simulink model "Nerthus_sim"  (R2021a)
settings: Solver=ode45  StartTime=0.0  StopTime=simtime  MaxStep=ts_max
values from neighbouring files (symbols this model uses):
  a_f = 1E-5*depl_fuel_temp_coef(depl_index)    [parameters.m]
  a_g = 1E-5*depl_grap_temp_coef(depl_index)    [parameters.m]
  A_s = 1.2245    [parameters.m]
  beta = depl_beta(depl_index,:)    [parameters.m]
  beta_t = sum(beta)    [parameters.m]
  Cp_1 = mean(interp1(Cal_temp1, Cal_Cp1, region_fdw))/1e3    [parameters.m]
  Cp_2 = mean(interp1(Cal_temp2, Cal_Cp2, region_sc))/1e3    [parameters.m]
  Cp_3 = mean(interp1(Cal_temp3, Cal_Cp3, region_s2))/1e3    [parameters.m]
  Cp_4 = mean(interp1(Cal_temp4, Cal_Cp4, region_s1))/1e3    [parameters.m]
  Cp_p = 0.00154912    [parameters.m]
  Cp_w = 456.056e-6    (= 0.000456056)    [parameters.m]
  D_it = 0.0141478    [parameters.m]
  D_ot = 0.015875    [parameters.m]
  DHRS_MODE = 1    [parameters.m]    (also in transients.m)
  DHRS_Power = P*(0.10)    (= 55.7)    [parameters.m]    (also in transients.m)
  DHRS_time = 20000000    [parameters.m]    (also in transients.m)
  DHRS_TIME_K = 10    [parameters.m]
  dHs_dPs = -0.042433622114357    (= -0.0424336221144)    [parameters.m]
  Epsilon = 1E-3    (= 0.001)    [parameters.m]
  Fiss_factor = 2.464783802008740e-03    (= 0.00246478380201)    [parameters.m]
  gamma0 = 9.635981959409105e-01    (= 0.963598195941)    [parameters.m]
  gamma1 = 3.560674858154914e-02    (= 0.0356067485815)    [parameters.m]
  gamma2 = 7.950554775404400e-04    (= 0.00079505547754)    [parameters.m]
  gamma_I = 5.1135e-2    (= 0.051135)    [parameters.m]
  gamma_Te = 6.1e-2    (= 0.061)    [parameters.m]
  gamma_Xe = 1.1628e-2    (= 0.011628)    [parameters.m]
  h_pw = h_s_shx    (= 0.00910134357894)    [parameters.m]
  H_s_table = zeros(m, n)    [parameters.m]
  h_wb = 13349.334646671E-6    (= 0.0133493346467)    [parameters.m]
  h_ws = 5732.378387768E-6    (= 0.00573237838777)    [parameters.m]
  h_wsc = 8385.005556375E-6    (= 0.00838500555638)    [parameters.m]
  hA_fg = 12.5325*SF_area_CORE    (= 12.5325)    [parameters.m]
  hA_p_phx1 = [UA_phx_nm,UA_phx_nm,UA_phx_nm,UA_phx_nm]    [parameters.m]
  hA_p_shx1 = [UA_shx_nm,UA_shx_nm,UA_shx_nm,UA_shx_nm]    [parameters.m]
  hA_s_phx1 = [UA_phx_nm,UA_phx_nm,UA_phx_nm,UA_phx_nm]    [parameters.m]
  hA_s_shx1 = [UA_shx_nm,UA_shx_nm,UA_shx_nm,UA_shx_nm]    [parameters.m]
  I_0 = ((gamma_I*Sig_f_msdr*phi_0) + (lam_Te*Te_0))/lam_I    (= 7.13664200441e+16)    [parameters.m]
  k_1 = 0.5    [parameters.m]
  K_1 = 11.632248097704855    (= 11.6322480977)    [parameters.m]
  k_2 = 0.5    [parameters.m]
  K_4 = b(1)    [parameters.m]
  K_5 = a(1)    [parameters.m]
  K_b = 12.834854076292217    (= 12.8348540763)    [parameters.m]
  k_f1 = k_f/nn_f    (= 0.465)    [parameters.m]
  k_f2 = k_f/nn_f    (= 0.465)    [parameters.m]
  k_g = 0.07    [parameters.m]
  K_pump = 10000000    [parameters.m]
  K_sc = -17.615718797133468    (= -17.6157187971)    [parameters.m]
  L = 8.5344*SF_length    (= 7.72866182253)    [parameters.m]
  L_b = 2.3645*SF_length    (= 2.14126603855)    [parameters.m]
  L_s = 4.723*SF_length    (= 4.27709854094)    [parameters.m]
  L_sc = 1.4469*SF_length    (= 1.31029724304)    [parameters.m]
  Lam = depl_Lam(depl_index)    [parameters.m]
  lam = [1.240E-02, 3.05E-02, 1.11E-01, 3.01E-01, 1.140E+00, 3.014E+00]    [parameters.m]
  lam_bubl = 2E-2    (= 0.02)    [parameters.m]
  lam_I = 2.875e-5    (= 2.875e-05)    [parameters.m]
  lam_Te = 3.65e-02    (= 0.0365)    [parameters.m]
  lam_Xe = 2.0916e-5    (= 2.0916e-05)    [parameters.m]
  lambda0 = 0.0945298    [parameters.m]
  lambda1 = 0.00441957    [parameters.m]
  lambda2 = 8.60979e-05    [parameters.m]
  m_f_t = mdot_fuel*(tau_core + tau_phx + tau_DHRS)    (= 116168.4)    [parameters.m]
  M_initial = L_b*rho_b*A_s + L_s*rho_s*A_s + L_sc*A_s*rho_sc    [parameters.m]
  M_stm = 0.018    [parameters.m]
  mcp_f1 = mn_f*scp_fuel    (= 62.07748875)    [parameters.m]
  mcp_f2 = mn_f*scp_fuel    (= 62.07748875)    [parameters.m]
  mcp_g1 = m_g*scp_graphite    (= 3731.2785)    [parameters.m]
  mcp_p_phx1 = scp_fuel*mp_phx1    [parameters.m]
  mcp_p_shx1 = scp_coolant*mp_shx1    [parameters.m]
  mcp_s_phx1 = scp_coolant*ms_phx1    [parameters.m]
  mcp_s_shx1 = scp_HITEC*ms_shx1    [parameters.m]
  mcp_t_phx1 = scp_tube*mt_phx1    [parameters.m]
  mcp_t_shx1 = scp_tube*mt_shx1    [parameters.m]
  mdot_coolant = 1543 + SF_fdw_PHX    (= 1543)    [parameters.m]
  mdot_HITEC = 3379 + SF_fdw_SHX    (= 3379)    [parameters.m]
  mn_f = (m_f/nn_f)    (= 31567.5)    [parameters.m]
  mn_piDHRS = mdot_fuel*tau_DHRS    (= 4209)    [parameters.m]
  mn_UHX = (tau_HITEC_UHX*mdot_HITEC)/n_UHX    (= 11263.3333333)    [parameters.m]
  mp_phx1 = [mp_phx_nm, mp_phx_nm, mp_phx_nm, mp_phx_nm]    [parameters.m]
  mp_shx1 = [mp_shx_nm, mp_shx_nm, mp_shx_nm, mp_shx_nm]    [parameters.m]
  ms_phx1 = [ms_phx_nm, ms_phx_nm, ms_phx_nm, ms_phx_nm]    [parameters.m]
  ms_shx1 = [ms_shx_nm, ms_shx_nm, ms_shx_nm, ms_shx_nm]    [parameters.m]
  N = 6546*SF_linear    (= 4861.496)    [parameters.m]
  n_frac0 = 1    [parameters.m]
  n_UHX = 3    [parameters.m]
  omega = 10.00000    (= 10)    [parameters.m]    (also in transients.m)
  P = 557    [parameters.m]    (also in transients.m)
  P_s = 12.5    [parameters.m]
  P_sat = 12.5    [parameters.m]
  P_sc = 12.5    [parameters.m]
  phi_0 = P/(3.04414e-17*1e6*Sig_f_msdr)    (= 3.1277117014e+14)    [parameters.m]
  Power_Bleed = P*(0.00)    (= 0)    [parameters.m]    (also in transients.m)
  pres_table = pres_inp    [parameters.m]
  R = 8.314462E-6    (= 8.314462e-06)    [parameters.m]
  rho_0 = beta_t - bterm    [parameters.m]
  rho_b = (XSteam('rho_pT', 125, 327.81) + XSteam('rho_pT', 125, 327.82))/2    [parameters.m]
  rho_p = rho_HITEC    (= 1680)    [parameters.m]
  rho_s = mean(interp1(Cal_temp_steam, Cal_rho3, region_steam))    [parameters.m]
  rho_sc = mean(interp1(Cal_temp2, Cal_rho2, region_sc))    [parameters.m]
  rho_w = 8425.712    [parameters.m]
  rhoXe_0 = (-sig_Xe / Sig_a) * (gamma_Te + gamma_I + gamma_Xe) * Sig_f_msdr * phi_0/(lam_Xe + sig_Xe * phi_0 + lam_bubl)    (= -0.000282704956487)    [parameters.m]
  scp_coolant = 8.83E-3    (= 0.00883)    [parameters.m]
  scp_fuel = 1.9665E-3    (= 0.0019665)    [parameters.m]
  scp_HITEC = 0.00154912    [parameters.m]
  Sig_f_msdr = U_den*U_sig    (= 0.058501076601)    [parameters.m]
  sig_Xe = 2.66449e-18    [parameters.m]
  sin_mag = 0    [parameters.m]    (also in transients.m)
  T0_f1 = Tf_in + (T0_f2-Tf_in)/2    (= 649.2)    [parameters.m]
  T0_f2 = 681.8    [parameters.m]
  T0_g1 = T0_f1 + (k_g*P/hA_fg)    (= 652.311111111)    [parameters.m]
  T0_p_phx1 = [663.1, 644.3, 630.3, 616.6]    [parameters.m]
  T0_p_shx1 = [641.8, 656.3, 621.4, 586.4]    [parameters.m]
  T0_s_phx1 = [595.1, 603.8, 615.6, 627.3]    [parameters.m]
  T0_s_shx1 = [598.2, 689.1, 651.4, 613.7]    [parameters.m]
  T0_t_phx1 = [639.3, 612.7]    [parameters.m]
  T0_t_shx1 = [646.6, 609.8]    [parameters.m]
  T_fw = 180.0    (= 180)    [parameters.m]
  T_p1 = 605.5    [parameters.m]
  T_p2 = 579.6    [parameters.m]
  T_p3 = 557.5    [parameters.m]
  ... (+40 more)
undefined symbols (not defined in the file or in its folder): C0, Cp_s, Cp_sc, ln, rho_f, scp_f, scp_s, vdot_f, vdot_s
libraries: pid_lib x1, simulink x1
(part 1 of 3)
settings Model: Creator=visura96  LastModifiedBy=visura96
settings SolverCC: AlgebraicLoopSolver=LineSearch
settings DataIOCC: ReturnWorkspaceOutputs=off
settings DebuggingCC: SFMachineParentedDataDiag=warning
settings SFSimCC: CustomCodeUndefinedFunction=UseInterfaceOnly

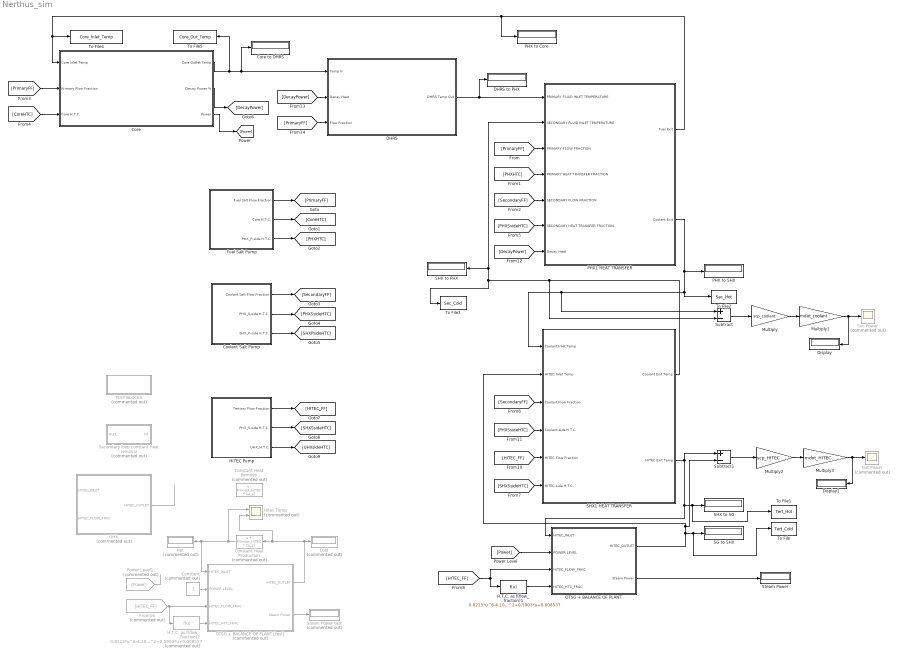
== system Nerthus_sim ==
  Cold : Display  Commented=on
  Constant : Constant  Commented=on
  Constant Heat Production : Fcn  Commented=on  Expr=u + P/(mdot_HITEC * Cp_p)
  Constant Heat Remove : Fcn  Commented=on  Expr=u - P/(mdot_HITEC * Cp_p)
  Coolant Salt Pump : Subsystem
  Core : Subsystem
  Core to DHRS : Display
  "DHRS " : Subsystem
  DHRS to PHX : Display
  Display : Display
  Display1 : Display
  From16 : From  Commented=on  GotoTag=HITEC_FF
  Fuel Salt Pump : Subsystem
  H.T.C. as f(flow_fraction)1 : Fcn  Expr=0.8215*u^6-4.108*u^5+7.848*u^4-7.165*u^3+3.004*u^2+0.5903*u+0.008537
  H.T.C. as f(flow_fraction)2 : Fcn  Commented=on  Expr=0.8215*u^6-4.108*u^5+7.848*u^4-7.165*u^3+3.004*u^2+0.5903*u+0.008537
  HITEC Pump : Subsystem
  Hitec Temp : Scope  Commented=on  NumInputPorts=2
  "Hot " : Display  Commented=on
  Multiply : Gain  Gain=scp_coolant
  Multiply1 : Gain  Gain=mdot_coolant
  Multiply2 : Gain  Gain=scp_HITEC
  Multiply3 : Gain  Gain=mdot_HITEC
  OTSG + BALANCE OF PLANT : Subsystem
  OTSG + BALANCE OF PLANT [test] : Subsystem  Commented=on
  PHX to Core : Display
  PHX to SHX : Display
  PHX1 HEAT TRANSFER : Subsystem
  Power Level1 : From  Commented=on  GotoTag=Power
  SG to SHX : Display
  SHX to PHX : Display
  SHX to SG : Display
  SHX1 HEAT TRANSFER : Subsystem
  Sec Power : Scope  Commented=on
  Secondary loop constant heat removal : Subsystem  Commented=on
  Steam Power : Display
  Steam Power test : Display  Commented=on
  Subtract : Sum  Inputs=+-
  Subtract1 : Sum  Inputs=+-
  TEST BLOCKS : Subsystem  Commented=on
  Tert Power : Scope  Commented=on
  To File : ToFile  Filename=Tert_Cold  MatrixName=Tert_Cold
  To File1 : ToFile  Filename=Tert_Hot  MatrixName=Tert_hot
  To File2 : ToFile  Filename=Sec_Hot  MatrixName=Sec_hot
  To File3 : ToFile  Filename=Sec_Cold  MatrixName=Sec_Cold
  To File4 : ToFile  Filename=Core_Inlet_Temp  MatrixName=Core_Inlet_Temp
  To File5 : ToFile  Filename=Core_Out_Temp  MatrixName=Core_Out_Temp
  UHX : Subsystem  Commented=on  VariantControl=UHX
  wires:
  Fuel Salt Pump/1(Fuel Salt Flow Fraction) -> [PrimaryFF]
  [PrimaryFF] -> Core/2(Primary Flow Fraction)
  Fuel Salt Pump/2(Core H.T.C.) -> [CoreHTC]
  [CoreHTC] -> Core/3(Core H.T.C.)
  Fuel Salt Pump/3(PHX_P-side H.T.C.) -> [PHXHTC]
  Coolant Salt Pump/1(Coolant Salt Flow Fraction) -> [SecondaryFF]
  Coolant Salt Pump/2(PHX_S-side H.T.C.) -> [PHXSsideHTC]
  Coolant Salt Pump/3(SHX_P-side H.T.C.) -> [SHXPsideHTC]
  Core/1(Core Outlet Temp) -> To File5/1, "DHRS "/1("Temp In "), Core to DHRS/1
  Core/2(Decay Power %) -> [DecayPower]
  HITEC Pump/2(PHX_S-side H.T.C.) -> [SHXSsideHTC]
  HITEC Pump/1(Tertiary Flow Fraction) -> [HITEC_FF]
  HITEC Pump/3(UHX_H.T.C.) -> [UHXsideHTC]
  [PrimaryFF] -> PHX1 HEAT TRANSFER/3(PRIMARY FLOW FRACTION)
  [PHXHTC] -> PHX1 HEAT TRANSFER/4(PRIMARY HEAT TRANSFER FRACTION)
  [SecondaryFF] -> PHX1 HEAT TRANSFER/5(SECONDARY FLOW FRACTION)
  [PHXSsideHTC] -> PHX1 HEAT TRANSFER/6(SECONDARY HEAT TRANSFER FRACTION)
  SHX1 HEAT TRANSFER/1(Coolant Exit Temp) -> Subtract/2, PHX1 HEAT TRANSFER/2(SECONDARY FLUID INLET TEMPERATURE), SHX to PHX/1, To File3/1
  PHX1 HEAT TRANSFER/2(Coolant Exit) -> To File2/1, Subtract/1, SHX1 HEAT TRANSFER/1(Coolant Inlet Temp), PHX to SHX/1
  [SecondaryFF] -> SHX1 HEAT TRANSFER/3(Coolant Flow Fraction)
  [SHXSsideHTC] -> SHX1 HEAT TRANSFER/6(HITEC-side H.T.C.)
  [HITEC_FF] -> SHX1 HEAT TRANSFER/5(HITEC Flow Fraction)
  [PHXSsideHTC] -> SHX1 HEAT TRANSFER/4(Coolant-side H.T.C.)
  [DecayPower] -> PHX1 HEAT TRANSFER/7(Decay Heat)
  "DHRS "/1("DHRS Temp Out ") -> DHRS to PHX/1, PHX1 HEAT TRANSFER/1(PRIMARY FLUID INLET TEMPERATURE)
  PHX1 HEAT TRANSFER/1(Fuel Exit) -> PHX to Core/1, Core/1("Core Inlet Temp "), To File4/1
  [DecayPower] -> "DHRS "/2(Decay Heat)
  [PrimaryFF] -> "DHRS "/3(Flow Fraction)
  UHX/1(HITEC_OUTLET) -> ?
  [HITEC_FF] -> OTSG + BALANCE OF PLANT/3(HITEC_FLOW_FRAC), H.T.C. as f(flow_fraction)1/1
  H.T.C. as f(flow_fraction)1/1 -> OTSG + BALANCE OF PLANT/4(HITEC_HTC_FRAC)
  Core/3(Power) -> [Power]
  Subtract/1 -> Multiply/1
  Multiply/1 -> Multiply1/1
  Multiply1/1 -> Display/1, Sec Power/1
  Multiply2/1 -> Multiply3/1
  Multiply3/1 -> Display1/1, Tert Power/1
  Subtract1/1 -> Multiply2/1
  Constant/1 -> OTSG + BALANCE OF PLANT [test]/2(POWER LEVEL)
  H.T.C. as f(flow_fraction)2/1 -> OTSG + BALANCE OF PLANT [test]/4(HITEC_HTC_FRAC)
  From16/1 -> H.T.C. as f(flow_fraction)2/1, OTSG + BALANCE OF PLANT [test]/3(HITEC_FLOW_FRAC)
  OTSG + BALANCE OF PLANT [test]/2(Steam Power) -> Steam Power test/1
  OTSG + BALANCE OF PLANT/2(Steam Power) -> Steam Power/1
  Power Level1/1 -> ?
  OTSG + BALANCE OF PLANT [test]/1(HITEC_OUTLET) -> Hitec Temp/2, Constant Heat Production/1, Cold/1
  Constant Heat Production/1 -> Hitec Temp/1, "Hot "/1, OTSG + BALANCE OF PLANT [test]/1(HITEC_INLET)
  [Power] -> OTSG + BALANCE OF PLANT/2(POWER LEVEL)
  SHX1 HEAT TRANSFER/2(HITEC Exit Temp) -> To File1/1, SHX to SG/1, OTSG + BALANCE OF PLANT/1(HITEC_INLET), Subtract1/1
  OTSG + BALANCE OF PLANT/1(HITEC_OUTLET) -> To File/1, SG to SHX/1, Subtract1/2, SHX1 HEAT TRANSFER/2(HITEC Inlet Temp)

== system Nerthus_sim/Coolant Salt Pump ==
  Clock1 : Clock
  Fcn : Fcn  Expr=(1-vdot_f_fc_pc)*exp(-K_pump*(u))+vdot_f_fc_pc
  PHX_S-side H.T.C. as f(flow_fraction) : Fcn  Expr=0.8215*u^6-4.108*u^5+7.848*u^4-7.165*u^3+3.004*u^2+0.5903*u+0.008537
  Pump Trip Time : TransportDelay  DelayTime=Trip_S_pump  BufferSize=4096
  SHX_P-side H.T.C. as f(flow_fraction) : Fcn  Expr=0.8215*u^6-4.108*u^5+7.848*u^4-7.165*u^3+3.004*u^2+0.5903*u+0.008537
  Scope : Scope
  Coolant Salt Flow Fraction : Outport  VectorParamsAs1DForOutWhenUnconnected=off
  PHX_S-side H.T.C. : Outport  Port=2  VectorParamsAs1DForOutWhenUnconnected=off
  SHX_P-side H.T.C. : Outport  Port=3  VectorParamsAs1DForOutWhenUnconnected=off
  wires:
  Fcn/1 -> SHX_P-side H.T.C. as f(flow_fraction)/1, PHX_S-side H.T.C. as f(flow_fraction)/1, Coolant Salt Flow Fraction/1, Scope/1
  Clock1/1 -> Pump Trip Time/1
  Pump Trip Time/1 -> Fcn/1
  PHX_S-side H.T.C. as f(flow_fraction)/1 -> PHX_S-side H.T.C./1
  SHX_P-side H.T.C. as f(flow_fraction)/1 -> SHX_P-side H.T.C./1

== system Nerthus_sim/Core ==
  "Core Inlet Temp " : Inport
  Primary Flow Fraction : Inport  Port=2
  Core H.T.C. : Inport  Port=3
  Core Heat Transfer : Subsystem
  Core to DHRS : VariableTransportDelay  MaximumDelay=10000000000  InitialOutput=T0_f2
  Decay Heat : Subsystem
  PKE SOLVER : Subsystem
  "Reactivity " : Subsystem
  tau_c_DHRS/PFF : Fcn  Expr=tau_core_DHRS/u
  Core Outlet Temp : Outport  VectorParamsAs1DForOutWhenUnconnected=off
  Decay Power % : Outport  Port=2  VectorParamsAs1DForOutWhenUnconnected=off
  Power : Outport  Port=3
  wires:
  "Core Inlet Temp "/1 -> Core Heat Transfer/3(Fuel In Temp)
  Primary Flow Fraction/1 -> tau_c_DHRS/PFF/1, PKE SOLVER/2(Primary Flow Fraction), Core Heat Transfer/5(Primary Flow Fraction)
  Core H.T.C./1 -> Core Heat Transfer/4(Core H.T.C.)
  Core Heat Transfer/1(Temp MUX) -> "Reactivity "/2(Temp MUX)
  PKE SOLVER/1((n/n_0)) -> Core Heat Transfer/1("(n/n_0) "), Decay Heat/1((n/n_0)), "Reactivity "/1((n/n_0))
  Core Heat Transfer/2(Fuel Out Temp) -> Core to DHRS/1
  tau_c_DHRS/PFF/1 -> Core to DHRS/2
  "Reactivity "/1(Reactivity Feed-back + Reactivity Additions) -> PKE SOLVER/1(Reactivity Feed-back + Reactivity Additions)
  Decay Heat/1("Relative Decay Power ") -> Core Heat Transfer/2(Decay Power %), Decay Power %/1
  Core to DHRS/1 -> Core Outlet Temp/1
  Core Heat Transfer/3(Power) -> Power/1

== system Nerthus_sim/DHRS  ==
  "Temp In " : Inport
  Decay Heat : Inport  Port=2
  Flow Fraction : Inport  Port=3
  Clock : Clock
  DHRS MODE : Constant  Value=DHRS_MODE
  DHRS to FP : VariableTransportDelay  MaximumDelay=10000000000  InitialOutput=T0_f2
  Integrator1 : Integrator  InitialCondition=T0_f2
  Mux : Mux  Inputs=6
      settings: DisplayOption=signals
  "NORNAML DHRS " : Fcn  Expr=(DHRS_Power-Power_Bleed)/(1+exp(ln(1/Epsilon - 1)*(1 - (u[6]-DHRS_time)/DHRS_TIME_K)))+Power_Bleed
  SLUG DATA : FromWorkspace  VariableName=slugger  SampleTime=1  Interpolate=off  OutputAfterFinalValue=Holding final value
  Scope1 : Scope
  Switch : Switch  Threshold=2
  To Workspace1 : ToWorkspace  VariableName=DHRS_outlet_temp  SampleTime=-1
  mn_piDHRS : Fcn  Expr="(u(3)*W_f/mn_piDHRS)*(u(1) - u(5)) - (u(4)/(mn_piDHRS*scp_fuel))  + (u(2)*P*mn_piDHRS/(m_f_t*scp_fuel*mn_piDHRS))"
  tau_DHRS_hx/PFF : Fcn  Expr=tau_DHRS_phx/u
  "DHRS Temp Out " : Outport  VectorParamsAs1DForOutWhenUnconnected=off
  wires:
  Mux/1 -> mn_piDHRS/1, "NORNAML DHRS "/1
  Flow Fraction/1 -> Mux/3, tau_DHRS_hx/PFF/1
  mn_piDHRS/1 -> Integrator1/1
  DHRS to FP/1 -> Scope1/1, To Workspace1/1, "DHRS Temp Out "/1
  tau_DHRS_hx/PFF/1 -> DHRS to FP/2
  Integrator1/1 -> Mux/5, DHRS to FP/1
  "Temp In "/1 -> Mux/1
  Decay Heat/1 -> Mux/2
  "NORNAML DHRS "/1 -> Switch/3
  SLUG DATA/1 -> Switch/1
  DHRS MODE/1 -> Switch/2
  Switch/1 -> Mux/4
  Clock/1 -> Mux/6

== system Nerthus_sim/Fuel Salt Pump ==
  Clock : Clock
  Core H.T.C. as f(flow_fraction) : Fcn  Expr=0.8215*u^6-4.108*u^5+7.848*u^4-7.165*u^3+3.004*u^2+0.5903*u+0.008537
  Display : Display
  Fcn : Fcn  Expr=(1-vdot_f_fc_pc)*exp(-K_pump*(u))+vdot_f_fc_pc
  PXH_P-side H.T.C. as f(flow_fraction) : Fcn  Expr=0.8215*u^6-4.108*u^5+7.848*u^4-7.165*u^3+3.004*u^2+0.5903*u+0.008537
  Pump Trip Time : TransportDelay  DelayTime=Trip_P_pump  BufferSize=4096
  Scope : Scope
  Fuel Salt Flow Fraction : Outport  VectorParamsAs1DForOutWhenUnconnected=off
  Core H.T.C. : Outport  Port=2  VectorParamsAs1DForOutWhenUnconnected=off
  PHX_P-side H.T.C. : Outport  Port=3  VectorParamsAs1DForOutWhenUnconnected=off
  wires:
  Fcn/1 -> Fuel Salt Flow Fraction/1, Scope/1, PXH_P-side H.T.C. as f(flow_fraction)/1, Core H.T.C. as f(flow_fraction)/1
  Clock/1 -> Pump Trip Time/1
  Pump Trip Time/1 -> Display/1, Fcn/1
  Core H.T.C. as f(flow_fraction)/1 -> Core H.T.C./1
  PXH_P-side H.T.C. as f(flow_fraction)/1 -> PHX_P-side H.T.C./1

== system Nerthus_sim/HITEC Pump ==
  Clock1 : Clock
  Fcn : Fcn  Expr=(1-vdot_f_fc_pc)*exp(-K_pump*(u))+vdot_f_fc_pc
  PHX_S-side H.T.C. as f(flow_fraction) : Fcn  Expr=0.8215*u^6-4.108*u^5+7.848*u^4-7.165*u^3+3.004*u^2+0.5903*u+0.008537
  Pump Trip Time : TransportDelay  DelayTime=Trip_T_pump  BufferSize=4096
  Radiator_S-side H.T.C. as f(flow_fraction) : Fcn  Expr=0.8215*u^6-4.108*u^5+7.848*u^4-7.165*u^3+3.004*u^2+0.5903*u+0.008537
  Scope : Scope
  Tertiary Flow Fraction : Outport  VectorParamsAs1DForOutWhenUnconnected=off
  PHX_S-side H.T.C. : Outport  Port=2  VectorParamsAs1DForOutWhenUnconnected=off
  UHX_H.T.C. : Outport  Port=3  VectorParamsAs1DForOutWhenUnconnected=off
  wires:
  Fcn/1 -> Radiator_S-side H.T.C. as f(flow_fraction)/1, PHX_S-side H.T.C. as f(flow_fraction)/1, Tertiary Flow Fraction/1, Scope/1
  Clock1/1 -> Pump Trip Time/1
  Pump Trip Time/1 -> Fcn/1
  PHX_S-side H.T.C. as f(flow_fraction)/1 -> PHX_S-side H.T.C./1
  Radiator_S-side H.T.C. as f(flow_fraction)/1 -> UHX_H.T.C./1

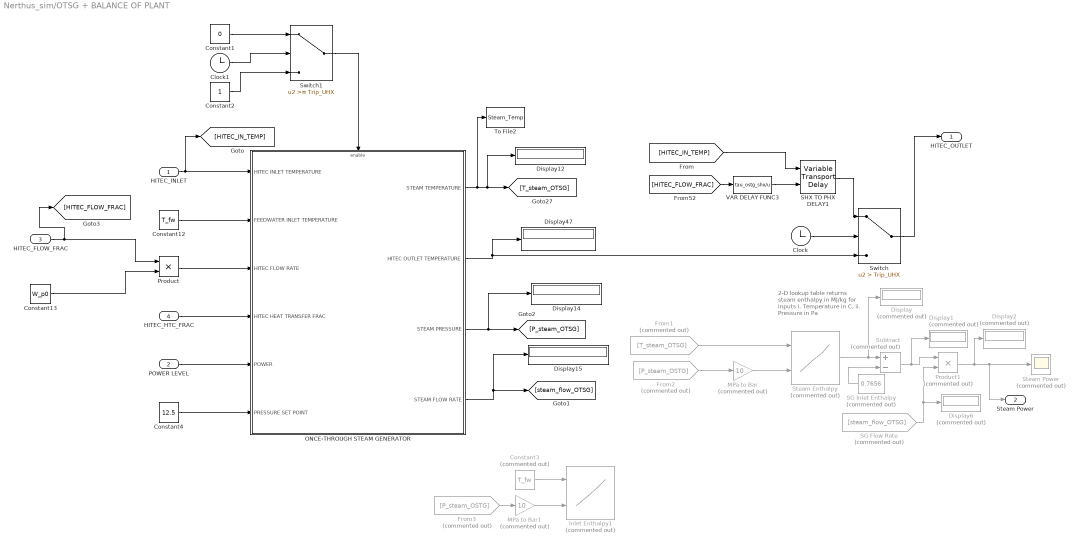
== system Nerthus_sim/OTSG + BALANCE OF PLANT ==
  note: 2-D lookup table returns steam enthalpy in MJ/kg for inputs i. Temperature in C, ii. Pressure in Pa
  HITEC_INLET : Inport
  POWER LEVEL : Inport  Port=2
  HITEC_FLOW_FRAC : Inport  Port=3
  HITEC_HTC_FRAC : Inport  Port=4
  Clock : Clock
  Clock1 : Clock
  Constant1 : Constant  Value=0
  Constant12 : Constant  Value=T_fw
  Constant13 : Constant  Value=W_p0
  Constant2 : Constant
  Constant3 : Constant  Commented=on  Value=T_fw
  Constant4 : Constant  Value=12.5
  Display{,1..2,6} (4 alike) : Display  Commented=on
  Display{12,14..15,47} (4 alike) : Display
  From1 : From  Commented=on  GotoTag=T_steam_OTSG
  From2 : From  Commented=on  GotoTag=P_steam_OSTG
  From3 : From  Commented=on  GotoTag=P_steam_OSTG
  Inlet Enthalpy1 : Lookup_n-D  Commented=on  BreakpointsForDimension1=temp_table  BreakpointsForDimension2=pres_table  Table=H_s_table  DiagnosticForOutOfRangeInput=Warning  InternalRulePriority=Speed  RndMeth=Simplest  InputSameDT=on
      settings: InputPortMap=u0,u1
  MPa to Bar : Gain  Commented=on  Gain=10
  MPa to Bar1 : Gain  Commented=on  Gain=10
  ONCE-THROUGH STEAM GENERATOR : Subsystem
  Product : Product
  Product1 : Product  Commented=on
  SG Flow Rate : From  Commented=on  GotoTag=steam_flow_OTSG
  "SG Inlet Enthalpy " : Constant  Commented=on  Value=0.7656
  SHX TO PHX DELAY1 : VariableTransportDelay  MaximumDelay=1000000000000  InitialOutput=570
  Steam Enthalpy : Lookup_n-D  Commented=on  BreakpointsForDimension1=temp_table  BreakpointsForDimension2=pres_table  Table=H_s_table  DiagnosticForOutOfRangeInput=Warning  InternalRulePriority=Speed  RndMeth=Simplest  InputSameDT=on
      settings: InputPortMap=u0,u1
  "Steam Power " : Scope  Commented=on
  Subtract : Sum  Commented=on  Inputs=+-
  Switch : Switch  Criteria=u2 > Threshold  Threshold=Trip_UHX
  Switch1 : Switch  Threshold=Trip_UHX
  To File2 : ToFile  Filename=Steam_Temp  MatrixName=Steam_Temp
  VAR DELAY FUNC3 : Fcn  Expr=tau_ostg_shx/u
  HITEC_OUTLET : Outport  VectorParamsAs1DForOutWhenUnconnected=off
  Steam Power : Outport  Port=2
  wires:
  ONCE-THROUGH STEAM GENERATOR/4(STEAM FLOW RATE) -> Display15/1, [steam_flow_OTSG]
  ONCE-THROUGH STEAM GENERATOR/2(HITEC OUTLET TEMPERATURE) -> Display47/1, Switch/3
  ONCE-THROUGH STEAM GENERATOR/1(STEAM TEMPERATURE) -> To File2/1, Display12/1, [T_steam_OTSG]
  ONCE-THROUGH STEAM GENERATOR/3(STEAM PRESSURE) -> Display14/1, [P_steam_OTSG]
  HITEC_INLET/1 -> ONCE-THROUGH STEAM GENERATOR/1(HITEC INLET TEMPERATURE), [HITEC_IN_TEMP]
  Constant4/1 -> ONCE-THROUGH STEAM GENERATOR/6(PRESSURE SET POINT)
  Constant12/1 -> ONCE-THROUGH STEAM GENERATOR/2(FEEDWATER INLET TEMPERATURE)
  HITEC_HTC_FRAC/1 -> ONCE-THROUGH STEAM GENERATOR/4(HITEC HEAT TRANSFER FRAC)
  Constant13/1 -> Product/2
  HITEC_FLOW_FRAC/1 -> Product/1, [HITEC_FLOW_FRAC]
  Product/1 -> ONCE-THROUGH STEAM GENERATOR/3(HITEC FLOW RATE)
  Switch/1 -> HITEC_OUTLET/1
  Clock/1 -> Switch/2
  [HITEC_FLOW_FRAC] -> VAR DELAY FUNC3/1
  [HITEC_IN_TEMP] -> SHX TO PHX DELAY1/1
  VAR DELAY FUNC3/1 -> SHX TO PHX DELAY1/2
  SHX TO PHX DELAY1/1 -> Switch/1
  Clock1/1 -> Switch1/2
  Constant1/1 -> Switch1/1
  Switch1/1 -> ONCE-THROUGH STEAM GENERATOR/Enable
  Constant2/1 -> Switch1/3
  Steam Enthalpy/1 -> Display/1, Subtract/1
  SG Flow Rate/1 -> Product1/2, Display6/1
  From2/1 -> MPa to Bar/1
  Product1/1 -> Display2/1, "Steam Power "/1, Steam Power/1
  Subtract/1 -> Display1/1, Product1/1
  From1/1 -> Steam Enthalpy/1
  "SG Inlet Enthalpy "/1 -> Subtract/2
  MPa to Bar/1 -> Steam Enthalpy/2
  POWER LEVEL/1 -> ONCE-THROUGH STEAM GENERATOR/5(POWER)
  From3/1 -> MPa to Bar1/1
  MPa to Bar1/1 -> Inlet Enthalpy1/2
  Constant3/1 -> Inlet Enthalpy1/1

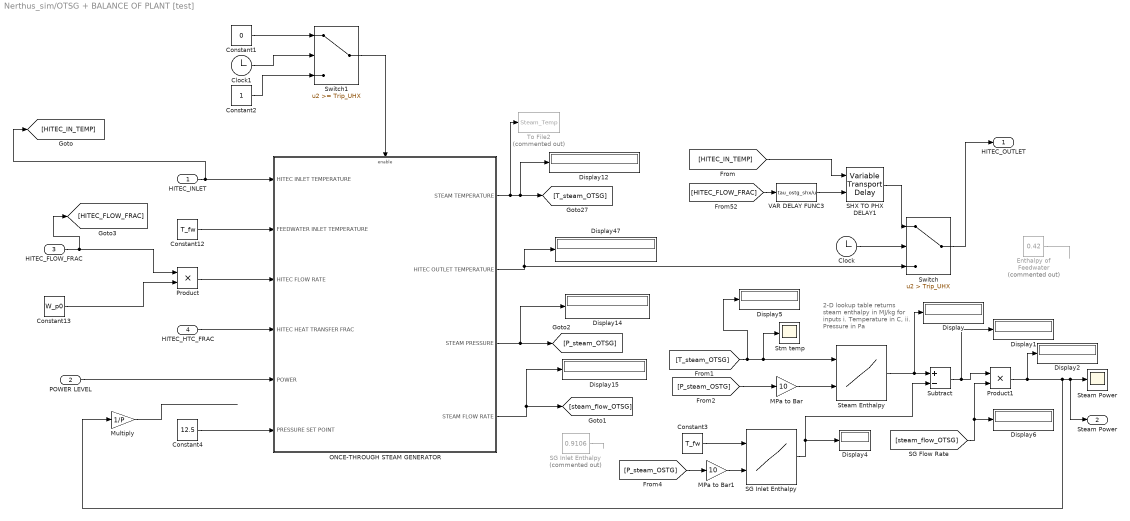
== system Nerthus_sim/OTSG + BALANCE OF PLANT [test] ==
  note: 2-D lookup table returns steam enthalpy in MJ/kg for inputs i. Temperature in C, ii. Pressure in Pa
  HITEC_INLET : Inport
  POWER LEVEL : Inport  Port=2
  HITEC_FLOW_FRAC : Inport  Port=3
  HITEC_HTC_FRAC : Inport  Port=4
  Clock : Clock
  Clock1 : Clock
  Constant1 : Constant  Value=0
  Constant12 : Constant  Value=T_fw
  Constant13 : Constant  Value=W_p0
  Constant2 : Constant
  Constant3 : Constant  Value=T_fw
  Constant4 : Constant  Value=12.5
  Display{,1..2,4..6,12,14..15,47} (10 alike) : Display
  Enthalpy of Feedwater : Constant  Commented=on  Value=0.42
  MPa to Bar : Gain  Gain=10
  MPa to Bar1 : Gain  Gain=10
  Multiply : Gain  Gain=1/P
  ONCE-THROUGH STEAM GENERATOR : Subsystem
  Product : Product
  Product1 : Product
  "SG Inlet Enthalpy " : Constant  Commented=on  Value=0.9106
  SG Inlet Enthalpy : Lookup_n-D  BreakpointsForDimension1=temp_table  BreakpointsForDimension2=pres_table  Table=H_s_table  DiagnosticForOutOfRangeInput=Warning  InternalRulePriority=Speed  RndMeth=Simplest  InputSameDT=on
      settings: InputPortMap=u0,u1
  SHX TO PHX DELAY1 : VariableTransportDelay  MaximumDelay=1000000000000  InitialOutput=570
  Steam Enthalpy : Lookup_n-D  BreakpointsForDimension1=temp_table  BreakpointsForDimension2=pres_table  Table=H_s_table  DiagnosticForOutOfRangeInput=Warning  InternalRulePriority=Speed  RndMeth=Simplest  InputSameDT=on
      settings: InputPortMap=u0,u1
  "Steam Power " : Scope
  Stm temp : Scope
  Subtract : Sum  Inputs=+-
  Switch : Switch  Criteria=u2 > Threshold  Threshold=Trip_UHX
  Switch1 : Switch  Threshold=Trip_UHX
  To File2 : ToFile  Commented=on  Filename=Steam_Temp  MatrixName=Steam_Temp
  VAR DELAY FUNC3 : Fcn  Expr=tau_ostg_shx/u
  HITEC_OUTLET : Outport  VectorParamsAs1DForOutWhenUnconnected=off
  Steam Power : Outport  Port=2
  wires:
  ONCE-THROUGH STEAM GENERATOR/4(STEAM FLOW RATE) -> Display15/1, [steam_flow_OTSG]
  ONCE-THROUGH STEAM GENERATOR/2(HITEC OUTLET TEMPERATURE) -> Display47/1, Switch/3
  ONCE-THROUGH STEAM GENERATOR/1(STEAM TEMPERATURE) -> To File2/1, Display12/1, [T_steam_OTSG]
  ONCE-THROUGH STEAM GENERATOR/3(STEAM PRESSURE) -> Display14/1, [P_steam_OTSG]
  HITEC_INLET/1 -> ONCE-THROUGH STEAM GENERATOR/1(HITEC INLET TEMPERATURE), [HITEC_IN_TEMP]
  Constant4/1 -> ONCE-THROUGH STEAM GENERATOR/6(PRESSURE SET POINT)
  Constant12/1 -> ONCE-THROUGH STEAM GENERATOR/2(FEEDWATER INLET TEMPERATURE)
  HITEC_HTC_FRAC/1 -> ONCE-THROUGH STEAM GENERATOR/4(HITEC HEAT TRANSFER FRAC)
  Constant13/1 -> Product/2
  HITEC_FLOW_FRAC/1 -> Product/1, [HITEC_FLOW_FRAC]
  Product/1 -> ONCE-THROUGH STEAM GENERATOR/3(HITEC FLOW RATE)
  Switch/1 -> HITEC_OUTLET/1
  Clock/1 -> Switch/2
  [HITEC_FLOW_FRAC] -> VAR DELAY FUNC3/1
  [HITEC_IN_TEMP] -> SHX TO PHX DELAY1/1
  VAR DELAY FUNC3/1 -> SHX TO PHX DELAY1/2
  SHX TO PHX DELAY1/1 -> Switch/1
  Clock1/1 -> Switch1/2
  Constant1/1 -> Switch1/1
  Switch1/1 -> ONCE-THROUGH STEAM GENERATOR/Enable
  Constant2/1 -> Switch1/3
  Steam Enthalpy/1 -> Subtract/1, Display/1
  [steam_flow_OTSG] -> Product1/2, Display6/1
  [P_steam_OSTG] -> MPa to Bar/1
  Product1/1 -> Display2/1, Multiply/1, Steam Power/1, "Steam Power "/1
  Subtract/1 -> Display1/1, Product1/1
  Enthalpy of Feedwater/1 -> ?
  [P_steam_OSTG] -> MPa to Bar1/1
  SG Inlet Enthalpy/1 -> Subtract/2, Display4/1
  [T_steam_OTSG] -> Stm temp/1, Steam Enthalpy/1, Display5/1
  Constant3/1 -> SG Inlet Enthalpy/1
  "SG Inlet Enthalpy "/1 -> ?
  MPa to Bar/1 -> Steam Enthalpy/2
  Multiply/1 -> ?
  POWER LEVEL/1 -> ONCE-THROUGH STEAM GENERATOR/5(POWER)
  MPa to Bar1/1 -> SG Inlet Enthalpy/2

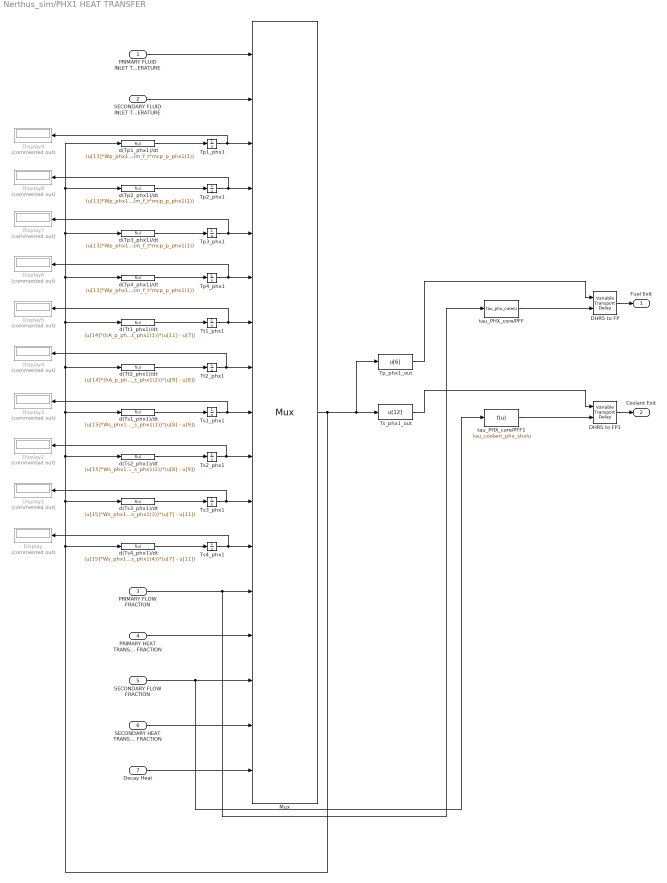
== system Nerthus_sim/PHX1 HEAT TRANSFER ==
  PRIMARY FLUID INLET TEMPERATURE : Inport
  SECONDARY FLUID INLET TEMPERATURE : Inport  Port=2
  PRIMARY FLOW FRACTION : Inport  Port=3
  PRIMARY HEAT TRANSFER FRACTION : Inport  Port=4
  SECONDARY FLOW FRACTION : Inport  Port=5
  SECONDARY HEAT TRANSFER FRACTION : Inport  Port=6
  Decay Heat : Inport  Port=7
  DHRS to FP : VariableTransportDelay  MaximumDelay=10000000000  InitialOutput=T0_p_phx1(4)
  DHRS to FP1 : VariableTransportDelay  MaximumDelay=10000000000  InitialOutput=T0_s_phx1(4)
  Display{,1..9} (10 alike) : Display  Commented=on
  Mux : Mux  Inputs=17
      settings: DisplayOption=signals
  Tp1_phx1 : Integrator  InitialCondition=T0_p_phx1(1)
  Tp2_phx1 : Integrator  InitialCondition=T0_p_phx1(2)
  "Tp3_phx1 " : Integrator  InitialCondition=T0_p_phx1(3)
  Tp4_phx1 : Integrator  InitialCondition=T0_p_phx1(4)
  Tp_phx1_out : Fcn  Expr=u[6]
  Ts1_phx1 : Integrator  InitialCondition=T0_s_phx1(1)
  Ts2_phx1 : Integrator  InitialCondition=T0_s_phx1(2)
  Ts3_phx1 : Integrator  InitialCondition=T0_s_phx1(3)
  Ts4_phx1 : Integrator  InitialCondition=T0_s_phx1(4)
  Ts_phx1_out : Fcn  Expr=u[12]
  Tt1_phx1 : Integrator  InitialCondition=T0_t_phx1(1)
  Tt2_phx1 : Integrator  InitialCondition=T0_t_phx1(2)
  d(Tp1_phx1)/dt : Fcn  Expr=(u[13]*Wp_phx1/mp_phx1(1))*(u[1] - u[3]) + (u[14]*hA_p_phx1(1)/mcp_p_phx1(1))*(u[7] - u[3]) + u(17)*P*mp_phx1(1)/(m_f_t*mcp_p_phx1(1))
  d(Tp2_phx1)/dt : Fcn  Expr=(u[13]*Wp_phx1/mp_phx1(2))*(u[3] - u[4]) + (u[14]*hA_p_phx1(2)/mcp_p_phx1(2))*(u[7] - u[3]) + u(17)*P*mp_phx1(1)/(m_f_t*mcp_p_phx1(1))
  d(Tp3_phx1)/dt : Fcn  Expr=(u[13]*Wp_phx1/mp_phx1(3))*(u[4] - u[5]) + (u[14]*hA_p_phx1(3)/mcp_p_phx1(3))*(u[8] - u[5]) + u(17)*P*mp_phx1(1)/(m_f_t*mcp_p_phx1(1))
  d(Tp4_phx1)/dt : Fcn  Expr=(u[13]*Wp_phx1/mp_phx1(4))*(u[5] - u[6]) + (u[14]*hA_p_phx1(4)/mcp_p_phx1(4))*(u[8] - u[5]) + u(17)*P*mp_phx1(1)/(m_f_t*mcp_p_phx1(1))
  d(Ts1_phx1)/dt : Fcn  Expr=(u[15]*Ws_phx1/ms_phx1(1))*(u[2] - u[9]) + (u[16]*hA_s_phx1(1)/mcp_s_phx1(1))*(u[8] - u[9])
  d(Ts2_phx1)/dt : Fcn  Expr=(u[15]*Ws_phx1/ms_phx1(2))*(u[9] - u[10]) + (u[16]*hA_s_phx1(2)/mcp_s_phx1(2))*(u[8] - u[9])
  d(Ts3_phx1)/dt : Fcn  Expr=(u[15]*Ws_phx1/ms_phx1(3))*(u[10] - u[11]) + (u[16]*hA_s_phx1(3)/mcp_s_phx1(3))*(u[7] - u[11])
  d(Ts4_phx1)/dt : Fcn  Expr=(u[15]*Ws_phx1/ms_phx1(4))*(u[11] - u[12]) + (u[16]*hA_s_phx1(4)/mcp_s_phx1(4))*(u[7] - u[11])
  d(Tt1_phx1)/dt : Fcn  Expr=(u[14]*(hA_p_phx1(1) + hA_p_phx1(2))/mcp_t_phx1(1))*(u[3] - u[7]) + (u[16]*(hA_s_phx1(1) + hA_s_phx1(2))/mcp_t_phx1(1))*(u[11] - u[7])
  d(Tt2_phx1)/dt : Fcn  Expr=(u[14]*(hA_p_phx1(3) + hA_p_phx1(4))/mcp_t_phx1(2))*(u[5] - u[8]) + (u[16]*(hA_s_phx1(3) + hA_s_phx1(4))/mcp_t_phx1(2))*(u[9] - u[8])
  tau_PHX_core/PFF : Fcn  Expr=tau_phx_core/u
  tau_PHX_core/PFF1 : Fcn  Expr=tau_coolant_phx_shx/u
  Fuel Exit : Outport  VectorParamsAs1DForOutWhenUnconnected=off
  Coolant Exit : Outport  Port=2  VectorParamsAs1DForOutWhenUnconnected=off
  wires:
  Ts1_phx1/1 -> Display3/1, Mux/9
  Ts2_phx1/1 -> Display2/1, Mux/10
  d(Ts2_phx1)/dt/1 -> Ts2_phx1/1
  d(Tp4_phx1)/dt/1 -> Tp4_phx1/1
  Tt1_phx1/1 -> Display5/1, Mux/7
  d(Tp2_phx1)/dt/1 -> Tp2_phx1/1
  Tp4_phx1/1 -> Display6/1, Mux/6
  d(Tt2_phx1)/dt/1 -> Tt2_phx1/1
  SECONDARY FLUID INLET TEMPERATURE/1 -> Mux/2
  Tt2_phx1/1 -> Display4/1, Mux/8
  d(Tp1_phx1)/dt/1 -> Tp1_phx1/1
  d(Ts4_phx1)/dt/1 -> Ts4_phx1/1
  Tp1_phx1/1 -> Display9/1, Mux/3
  d(Ts1_phx1)/dt/1 -> Ts1_phx1/1
  d(Ts3_phx1)/dt/1 -> Ts3_phx1/1
  Ts3_phx1/1 -> Display1/1, Mux/11
  Ts4_phx1/1 -> Display/1, Mux/12
  "Tp3_phx1 "/1 -> Display7/1, Mux/5
  d(Tp3_phx1)/dt/1 -> "Tp3_phx1 "/1
  Tp2_phx1/1 -> Display8/1, Mux/4
  d(Tt1_phx1)/dt/1 -> Tt1_phx1/1
  PRIMARY FLUID INLET TEMPERATURE/1 -> Mux/1
  PRIMARY FLOW FRACTION/1 -> tau_PHX_core/PFF/1, Mux/13
  PRIMARY HEAT TRANSFER FRACTION/1 -> Mux/14
  SECONDARY HEAT TRANSFER FRACTION/1 -> Mux/16
  SECONDARY FLOW FRACTION/1 -> tau_PHX_core/PFF1/1, Mux/15
  Decay Heat/1 -> Mux/17
  Mux/1 -> Ts_phx1_out/1, Tp_phx1_out/1, d(Ts4_phx1)/dt/1, d(Ts3_phx1)/dt/1, d(Ts1_phx1)/dt/1, d(Tt2_phx1)/dt/1, d(Tt1_phx1)/dt/1, d(Tp4_phx1)/dt/1, d(Tp3_phx1)/dt/1, d(Tp2_phx1)/dt/1, d(Tp1_phx1)/dt/1, d(Ts2_phx1)/dt/1
  tau_PHX_core/PFF/1 -> DHRS to FP/2
  Tp_phx1_out/1 -> DHRS to FP/1
  DHRS to FP/1 -> Fuel Exit/1
  tau_PHX_core/PFF1/1 -> DHRS to FP1/2
  Ts_phx1_out/1 -> DHRS to FP1/1
  DHRS to FP1/1 -> Coolant Exit/1

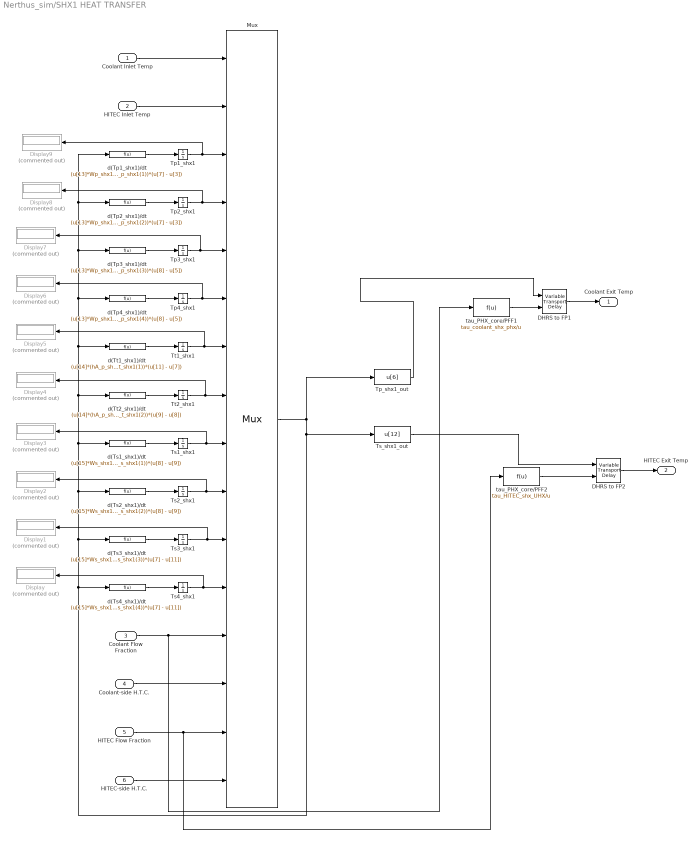
== system Nerthus_sim/SHX1 HEAT TRANSFER ==
  Coolant Inlet Temp : Inport
  HITEC Inlet Temp : Inport  Port=2
  Coolant Flow Fraction : Inport  Port=3
  Coolant-side H.T.C. : Inport  Port=4
  HITEC Flow Fraction : Inport  Port=5
  HITEC-side H.T.C. : Inport  Port=6
  DHRS to FP1 : VariableTransportDelay  MaximumDelay=10000000000  InitialOutput=T0_p_shx1(4)
  DHRS to FP2 : VariableTransportDelay  MaximumDelay=10000000000  InitialOutput=T0_s_shx1(4)
  Display{,1..9} (10 alike) : Display  Commented=on
  Mux : Mux  Inputs=16
      settings: DisplayOption=signals
  Tp1_shx1 : Integrator  InitialCondition=T0_p_shx1(1)
  Tp2_shx1 : Integrator  InitialCondition=T0_p_shx1(2)
  "Tp3_shx1 " : Integrator  InitialCondition=T0_p_shx1(3)
  Tp4_shx1 : Integrator  InitialCondition=T0_p_shx1(4)
  Tp_shx1_out : Fcn  Expr=u[6]
  Ts1_shx1 : Integrator  InitialCondition=T0_s_shx1(1)
  Ts2_shx1 : Integrator  InitialCondition=T0_s_shx1(2)
  Ts3_shx1 : Integrator  InitialCondition=T0_s_shx1(3)
  Ts4_shx1 : Integrator  InitialCondition=T0_s_shx1(4)
  Ts_shx1_out : Fcn  Expr=u[12]
  Tt1_shx1 : Integrator  InitialCondition=T0_t_shx1(1)
  Tt2_shx1 : Integrator  InitialCondition=T0_t_shx1(2)
  d(Tp1_shx1)/dt : Fcn  Expr=(u[13]*Wp_shx1/mp_shx1(1))*(u[1] - u[3]) + (u[14]*hA_p_shx1(1)/mcp_p_shx1(1))*(u[7] - u[3])
  d(Tp2_shx1)/dt : Fcn  Expr=(u[13]*Wp_shx1/mp_shx1(2))*(u[3] - u[4]) + (u[14]*hA_p_shx1(2)/mcp_p_shx1(2))*(u[7] - u[3])
  d(Tp3_shx1)/dt : Fcn  Expr=(u[13]*Wp_shx1/mp_shx1(3))*(u[4] - u[5]) + (u[14]*hA_p_shx1(3)/mcp_p_shx1(3))*(u[8] - u[5])
  d(Tp4_shx1)/dt : Fcn  Expr=(u[13]*Wp_shx1/mp_shx1(4))*(u[5] - u[6]) + (u[14]*hA_p_shx1(4)/mcp_p_shx1(4))*(u[8] - u[5])
  d(Ts1_shx1)/dt : Fcn  Expr=(u[15]*Ws_shx1/ms_shx1(1))*(u[2] - u[9]) + (u[16]*hA_s_shx1(1)/mcp_s_shx1(1))*(u[8] - u[9])
  d(Ts2_shx1)/dt : Fcn  Expr=(u[15]*Ws_shx1/ms_shx1(2))*(u[9] - u[10]) + (u[16]*hA_s_shx1(2)/mcp_s_shx1(2))*(u[8] - u[9])
  d(Ts3_shx1)/dt : Fcn  Expr=(u[15]*Ws_shx1/ms_shx1(3))*(u[10] - u[11]) + (u[16]*hA_s_shx1(3)/mcp_s_shx1(3))*(u[7] - u[11])
  d(Ts4_shx1)/dt : Fcn  Expr=(u[15]*Ws_shx1/ms_shx1(4))*(u[11] - u[12]) + (u[16]*hA_s_shx1(4)/mcp_s_shx1(4))*(u[7] - u[11])
  d(Tt1_shx1)/dt : Fcn  Expr=(u[14]*(hA_p_shx1(1) + hA_p_shx1(2))/mcp_t_shx1(1))*(u[3] - u[7]) + (u[16]*(hA_s_shx1(1) + hA_s_shx1(2))/mcp_t_shx1(1))*(u[11] - u[7])
  d(Tt2_shx1)/dt : Fcn  Expr=(u[14]*(hA_p_shx1(3) + hA_p_shx1(4))/mcp_t_shx1(2))*(u[5] - u[8]) + (u[16]*(hA_s_shx1(3) + hA_s_shx1(4))/mcp_t_shx1(2))*(u[9] - u[8])
  tau_PHX_core/PFF1 : Fcn  Expr=tau_coolant_shx_phx/u
  tau_PHX_core/PFF2 : Fcn  Expr=tau_HITEC_shx_UHX/u
  Coolant Exit Temp : Outport  VectorParamsAs1DForOutWhenUnconnected=off
  HITEC Exit Temp : Outport  Port=2  VectorParamsAs1DForOutWhenUnconnected=off
  wires:
  d(Ts2_shx1)/dt/1 -> Ts2_shx1/1
  d(Tp4_shx1)/dt/1 -> Tp4_shx1/1
  Tt1_shx1/1 -> Display5/1, Mux/7
  d(Tp2_shx1)/dt/1 -> Tp2_shx1/1
  Tp4_shx1/1 -> Display6/1, Mux/6
  d(Tt2_shx1)/dt/1 -> Tt2_shx1/1
  HITEC Inlet Temp/1 -> Mux/2
  Tt2_shx1/1 -> Display4/1, Mux/8
  Mux/1 -> Tp_shx1_out/1, Ts_shx1_out/1, d(Ts4_shx1)/dt/1, d(Ts3_shx1)/dt/1, d(Ts2_shx1)/dt/1, d(Ts1_shx1)/dt/1, d(Tt2_shx1)/dt/1, d(Tt1_shx1)/dt/1, d(Tp4_shx1)/dt/1, d(Tp3_shx1)/dt/1, d(Tp2_shx1)/dt/1, d(Tp1_shx1)/dt/1
  d(Tp1_shx1)/dt/1 -> Tp1_shx1/1
  d(Ts4_shx1)/dt/1 -> Ts4_shx1/1
  d(Ts1_shx1)/dt/1 -> Ts1_shx1/1
  d(Ts3_shx1)/dt/1 -> Ts3_shx1/1
  Ts3_shx1/1 -> Display1/1, Mux/11
  Ts4_shx1/1 -> Display/1, Mux/12
  "Tp3_shx1 "/1 -> Display7/1, Mux/5
  d(Tp3_shx1)/dt/1 -> "Tp3_shx1 "/1
  d(Tt1_shx1)/dt/1 -> Tt1_shx1/1
  Coolant Inlet Temp/1 -> Mux/1
  Coolant-side H.T.C./1 -> Mux/14
  HITEC-side H.T.C./1 -> Mux/16
  Coolant Flow Fraction/1 -> tau_PHX_core/PFF1/1, Mux/13
  HITEC Flow Fraction/1 -> tau_PHX_core/PFF2/1, Mux/15
  tau_PHX_core/PFF1/1 -> DHRS to FP1/2
  Tp_shx1_out/1 -> DHRS to FP1/1
  DHRS to FP1/1 -> Coolant Exit Temp/1
  Ts_shx1_out/1 -> DHRS to FP2/1
  tau_PHX_core/PFF2/1 -> DHRS to FP2/2
  DHRS to FP2/1 -> HITEC Exit Temp/1
  Ts1_shx1/1 -> Display3/1, Mux/9
  Ts2_shx1/1 -> Display2/1, Mux/10
  Tp1_shx1/1 -> Display9/1, Mux/3
  Tp2_shx1/1 -> Display8/1, Mux/4

== system Nerthus_sim/Secondary loop constant heat removal ==
  In1 : Inport
  Fcn : Fcn  Expr=u(1) - 500/(mdot_HITEC*scp_HITEC)
  Mux : Mux  Inputs=2
  Out1 : Outport  VectorParamsAs1DForOutWhenUnconnected=off
  wires:
  In1/1 -> Mux/1
  Fcn/1 -> Out1/1, Mux/2
  Mux/1 -> Fcn/1

== system Nerthus_sim/TEST BLOCKS ==
  Primary loop constant heat production : Subsystem  Commented=through
  Primary loop constant heat removal : Subsystem  Commented=through
  Secondaary loop constant heat production : Subsystem  Commented=through
  Secondary loop constant heat removal : Subsystem  Commented=through

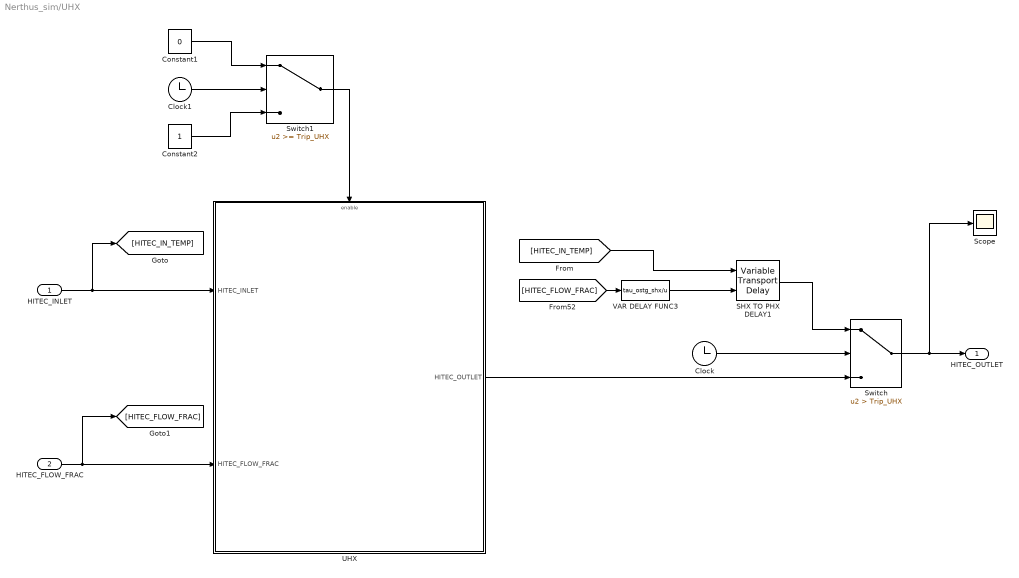
== system Nerthus_sim/UHX ==
  HITEC_INLET : Inport
  HITEC_FLOW_FRAC : Inport  Port=2
  Clock : Clock
  Clock1 : Clock
  Constant1 : Constant  Value=0
  Constant2 : Constant
  SHX TO PHX DELAY1 : VariableTransportDelay  MaximumDelay=1000000000000  InitialOutput=T0_s_shx1(1)
  Scope : Scope
  Switch : Switch  Criteria=u2 > Threshold  Threshold=Trip_UHX
  Switch1 : Switch  Threshold=Trip_UHX
  UHX : Subsystem
  VAR DELAY FUNC3 : Fcn  Expr=tau_ostg_shx/u
  HITEC_OUTLET : Outport  VectorParamsAs1DForOutWhenUnconnected=off
  wires:
  HITEC_FLOW_FRAC/1 -> [HITEC_FLOW_FRAC], UHX/2(HITEC_FLOW_FRAC)
  HITEC_INLET/1 -> [HITEC_IN_TEMP], UHX/1(HITEC_INLET)
  Switch/1 -> Scope/1, HITEC_OUTLET/1
  Clock/1 -> Switch/2
  [HITEC_FLOW_FRAC] -> VAR DELAY FUNC3/1
  UHX/1(HITEC_OUTLET) -> Switch/3
  VAR DELAY FUNC3/1 -> SHX TO PHX DELAY1/2
  SHX TO PHX DELAY1/1 -> Switch/1
  [HITEC_IN_TEMP] -> SHX TO PHX DELAY1/1
  Constant1/1 -> Switch1/1
  Constant2/1 -> Switch1/3
  Switch1/1 -> UHX/Enable
  Clock1/1 -> Switch1/2

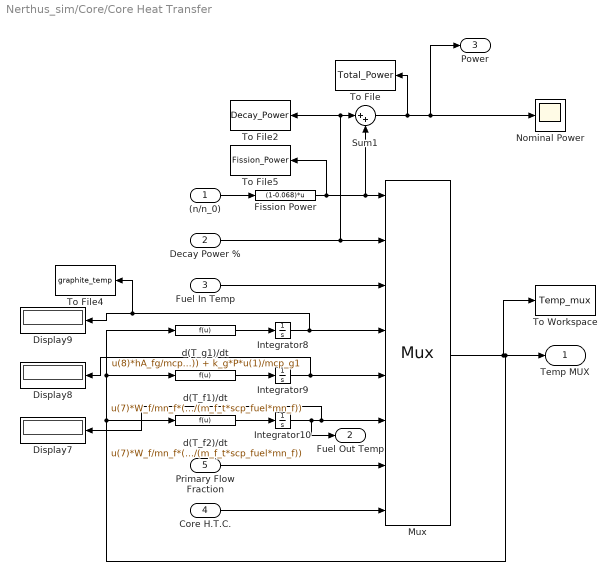
== system Nerthus_sim/Core/Core Heat Transfer ==
  "(n/n_0) " : Inport
  Decay Power % : Inport  Port=2
  Fuel In Temp : Inport  Port=3
  Core H.T.C. : Inport  Port=4
  Primary Flow Fraction : Inport  Port=5
  Display7 : Display
  Display8 : Display
  Display9 : Display
  Fission Power : Fcn  Expr=(1-0.068)*u
  Integrator10 : Integrator  InitialCondition=T0_f2
  Integrator8 : Integrator  InitialCondition=T0_g1
  Integrator9 : Integrator  InitialCondition=T0_f1
  Mux : Mux  Inputs=8
      settings: DisplayOption=signals
  Nominal Power : Scope
  Sum1 : Sum  Inputs=|++
  To File : ToFile  Filename=Total_Power  MatrixName=Total_Power
  To File2 : ToFile  Filename=Decay_Power  MatrixName=Decay_Power
  To File4 : ToFile  Filename=graphite_temp  MatrixName=graphite_temp
  To File5 : ToFile  Filename=Fission_Power  MatrixName=Fission_Power
  To Workspace : ToWorkspace  VariableName=Temp_mux  SampleTime=-1
  d(T_f1)/dt : Fcn  Expr=u(7)*W_f/mn_f*(u(3) - u(5)) + (k_f1*P*u(1)/mcp_f1) + (u(8)*hA_fg*k_1*(u(4) - u(5))/mcp_f1) + (u(2)*P*mn_f/(m_f_t*scp_fuel*mn_f))
  d(T_f2)/dt : Fcn  Expr="u(7)*W_f/mn_f*(u(5) - u(6)) + (k_f2*P*u(1)/mcp_f2) + (u(8)*hA_fg*k_2*(u(4) - u(5))/mcp_f2)  + (u(2)*P*mn_f/(m_f_t*scp_fuel*mn_f))"
  d(T_g1)/dt : Fcn  Expr=u(8)*hA_fg/mcp_g1*(u(5) - u(4)) + k_g*P*u(1)/mcp_g1
  Temp MUX : Outport  VectorParamsAs1DForOutWhenUnconnected=off
  Fuel Out Temp : Outport  Port=2  VectorParamsAs1DForOutWhenUnconnected=off
  Power : Outport  Port=3
  wires:
  d(T_g1)/dt/1 -> Integrator8/1
  d(T_f1)/dt/1 -> Integrator9/1
  d(T_f2)/dt/1 -> Integrator10/1
  Integrator10/1 -> Fuel Out Temp/1, Display7/1, Mux/6
  Integrator9/1 -> Display8/1, Mux/5
  Integrator8/1 -> To File4/1, Display9/1, Mux/4
  Mux/1 -> To Workspace/1, d(T_g1)/dt/1, d(T_f1)/dt/1, d(T_f2)/dt/1, Temp MUX/1
  Decay Power %/1 -> Sum1/1, To File2/1, Mux/2
  Fuel In Temp/1 -> Mux/3
  "(n/n_0) "/1 -> Fission Power/1
  Fission Power/1 -> To File5/1, Mux/1, Sum1/2
  Primary Flow Fraction/1 -> Mux/7
  Core H.T.C./1 -> Mux/8
  Sum1/1 -> To File/1, Power/1, Nominal Power/1

== system Nerthus_sim/Core/Decay Heat ==
  (n/n_0) : Inport
  Decay Power Percentage : Fcn  Expr=u(2)+u(3)+u(4)
  Decay Precursor G1 : Fcn  Expr=u(1)*Fiss_factor*gamma0 - lambda0*u(2)
  Decay Precursor G2 : Fcn  Expr=u(1)*Fiss_factor*gamma1 - lambda1*u(3)
  Decay Precursor G3 : Fcn  Expr=u(1)*Fiss_factor*gamma2 - lambda2*u(4)
  Integrator : Integrator  InitialCondition=0.025125
  Integrator1 : Integrator  InitialCondition=0.0198578
  Integrator2 : Integrator  InitialCondition=0.0227606
  Mux : Mux
      settings: DisplayOption=signals
  Scope : Scope
  To Workspace : ToWorkspace  VariableName=Decay_Group_total  SampleTime=-1
  To Workspace1 : ToWorkspace  VariableName=Decay_Groups1  SampleTime=-1
  To Workspace2 : ToWorkspace  VariableName=Decay_Groups2  SampleTime=-1
  To Workspace3 : ToWorkspace  VariableName=Decay_Groups3  SampleTime=-1
  "Relative Decay Power " : Outport  VectorParamsAs1DForOutWhenUnconnected=off
  wires:
  Decay Power Percentage/1 -> "Relative Decay Power "/1, Scope/1, To Workspace/1
  Decay Precursor G1/1 -> Integrator/1
  Decay Precursor G2/1 -> Integrator1/1
  Decay Precursor G3/1 -> Integrator2/1
  Mux/1 -> Decay Precursor G3/1, Decay Precursor G2/1, Decay Precursor G1/1, Decay Power Percentage/1
  Integrator/1 -> Mux/2, To Workspace1/1
  Integrator1/1 -> Mux/3, To Workspace2/1
  Integrator2/1 -> Mux/4, To Workspace3/1
  (n/n_0)/1 -> Mux/1

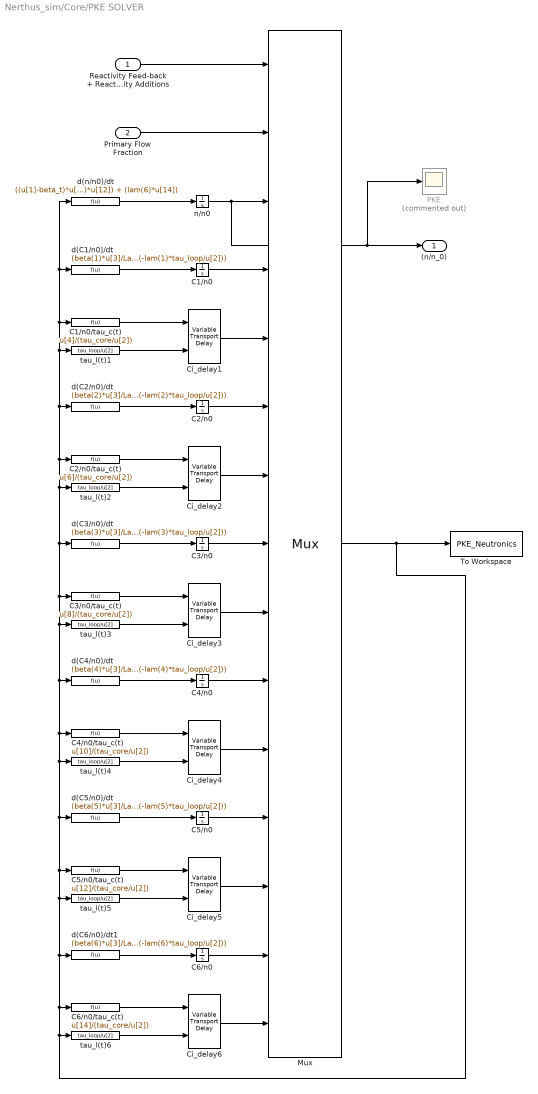
== system Nerthus_sim/Core/PKE SOLVER ==
  Reactivity Feed-back + Reactivity Additions : Inport
  Primary Flow Fraction : Inport  Port=2
  C1/n0 : Integrator  InitialCondition=C0(1)
  C1/n0/tau_c(t) : Fcn  Expr=u[4]/(tau_core/u[2])
  C2/n0 : Integrator  InitialCondition=C0(2)
  C2/n0/tau_c(t) : Fcn  Expr=u[6]/(tau_core/u[2])
  C3/n0 : Integrator  InitialCondition=C0(3)
  C3/n0/tau_c(t) : Fcn  Expr=u[8]/(tau_core/u[2])
  C4/n0 : Integrator  InitialCondition=C0(4)
  C4/n0/tau_c(t) : Fcn  Expr=u[10]/(tau_core/u[2])
  C5/n0 : Integrator  InitialCondition=C0(5)
  C5/n0/tau_c(t) : Fcn  Expr=u[12]/(tau_core/u[2])
  C6/n0 : Integrator  InitialCondition=C0(6)
  C6/n0/tau_c(t) : Fcn  Expr=u[14]/(tau_core/u[2])
  Ci_delay1 : VariableTransportDelay  MaximumDelay=10000000000  InitialOutput=C0(1)/tau_core
  Ci_delay2 : VariableTransportDelay  MaximumDelay=10000000000  InitialOutput=C0(2)/tau_core
  Ci_delay3 : VariableTransportDelay  MaximumDelay=10000000000  InitialOutput=C0(3)/tau_core
  Ci_delay4 : VariableTransportDelay  MaximumDelay=10000000000000  InitialOutput=C0(4)/tau_core
  Ci_delay5 : VariableTransportDelay  MaximumDelay=10000000000  InitialOutput=C0(5)/tau_core
  Ci_delay6 : VariableTransportDelay  MaximumDelay=10000000000000  InitialOutput=C0(6)/tau_core
  Mux : Mux  Inputs=15
      settings: DisplayOption=signals
  PKE : Scope  Commented=on
  To Workspace : ToWorkspace  VariableName=PKE_Neutronics  SampleTime=-1
  d(C1/n0)/dt : Fcn  Expr=(beta(1)*u[3]/Lam) - (lam(1)*u[4]) - (u[4]/(tau_core/u[2])) + (u[5]*exp(-lam(1)*tau_loop/u[2]))
  d(C2/n0)/dt : Fcn  Expr=(beta(2)*u[3]/Lam) - (lam(2)*u[6]) - (u[6]/(tau_core/u[2])) + (u[7]*exp(-lam(2)*tau_loop/u[2]))
  d(C3/n0)/dt : Fcn  Expr=(beta(3)*u[3]/Lam) - (lam(3)*u[8]) - (u[8]/(tau_core/u[2])) + (u[9]*exp(-lam(3)*tau_loop/u[2]))
  d(C4/n0)/dt : Fcn  Expr=(beta(4)*u[3]/Lam) - (lam(4)*u[10]) - (u[10]/(tau_core/u[2])) + (u[11]*exp(-lam(4)*tau_loop/u[2]))
  d(C5/n0)/dt : Fcn  Expr=(beta(5)*u[3]/Lam) - (lam(5)*u[12]) - (u[12]/(tau_core/u[2])) + (u[13]*exp(-lam(5)*tau_loop/u[2]))
  d(C6/n0)/dt1 : Fcn  Expr=(beta(6)*u[3]/Lam) - (lam(6)*u[14]) - (u[14]/(tau_core/u[2])) + (u[14]*exp(-lam(6)*tau_loop/u[2]))
  d(n/n0)/dt : Fcn  Expr=((u[1]-beta_t)*u[3]/Lam) + (lam(1)*u[4]) + (lam(2)*u[6]) + (lam(3)*u[8]) + (lam(4)*u[10]) + (lam(5)*u[12]) + (lam(6)*u[14])
  n/n0 : Integrator  InitialCondition=n_frac0
  tau_l(t){1..6} (6 alike) : Fcn  Expr=tau_loop/u[2]
  (n/n_0) : Outport  VectorParamsAs1DForOutWhenUnconnected=off
  wires:
  C1/n0/tau_c(t)/1 -> Ci_delay1/1
  d(n/n0)/dt/1 -> n/n0/1
  d(C1/n0)/dt/1 -> C1/n0/1
  Reactivity Feed-back + Reactivity Additions/1 -> Mux/1
  n/n0/1 -> (n/n_0)/1, PKE/1, Mux/3
  Primary Flow Fraction/1 -> Mux/2
  C1/n0/1 -> Mux/4
  Ci_delay1/1 -> Mux/5
  tau_l(t)1/1 -> Ci_delay1/2
  C2/n0/tau_c(t)/1 -> Ci_delay2/1
  d(C2/n0)/dt/1 -> C2/n0/1
  tau_l(t)2/1 -> Ci_delay2/2
  Ci_delay2/1 -> Mux/7
  C2/n0/1 -> Mux/6
  C3/n0/1 -> Mux/8
  d(C3/n0)/dt/1 -> C3/n0/1
  tau_l(t)3/1 -> Ci_delay3/2
  Ci_delay3/1 -> Mux/9
  C3/n0/tau_c(t)/1 -> Ci_delay3/1
  C4/n0/1 -> Mux/10
  C4/n0/tau_c(t)/1 -> Ci_delay4/1
  tau_l(t)4/1 -> Ci_delay4/2
  d(C4/n0)/dt/1 -> C4/n0/1
  Ci_delay4/1 -> Mux/11
  C5/n0/tau_c(t)/1 -> Ci_delay5/1
  d(C5/n0)/dt/1 -> C5/n0/1
  tau_l(t)5/1 -> Ci_delay5/2
  C5/n0/1 -> Mux/12
  Ci_delay5/1 -> Mux/13
  C6/n0/1 -> Mux/14
  tau_l(t)6/1 -> Ci_delay6/2
  d(C6/n0)/dt1/1 -> C6/n0/1
  C6/n0/tau_c(t)/1 -> Ci_delay6/1
  Ci_delay6/1 -> Mux/15
  Mux/1 -> To Workspace/1, tau_l(t)4/1, d(n/n0)/dt/1, d(C1/n0)/dt/1, C1/n0/tau_c(t)/1, tau_l(t)1/1, d(C2/n0)/dt/1, C2/n0/tau_c(t)/1, tau_l(t)2/1, d(C3/n0)/dt/1, C3/n0/tau_c(t)/1, tau_l(t)3/1, d(C4/n0)/dt/1, C4/n0/tau_c(t)/1, d(C5/n0)/dt/1, C5/n0/tau_c(t)/1, tau_l(t)5/1, d(C6/n0)/dt1/1, C6/n0/tau_c(t)/1, tau_l(t)6/1

== system Nerthus_sim/Core/Reactivity  ==
  (n/n_0) : Inport
  Temp MUX : Inport  Port=2
  Temp + Reactity Insertions : Subsystem
  Xe Reactivity : Subsystem
  Xe Reactivity Old : Subsystem  Commented=on
  Xe Reactivity1 : Subsystem  Commented=on
  Xe_Reactivity : Scope
  Reactivity Feed-back + Reactivity Additions : Outport  VectorParamsAs1DForOutWhenUnconnected=off
  wires:
  Temp MUX/1 -> Temp + Reactity Insertions/1("Temp MUX ")
  Temp + Reactity Insertions/1(Reactivity Feedback) -> Reactivity Feed-back + Reactivity Additions/1
  Xe Reactivity/1(drho_Xe) -> Xe_Reactivity/1, Temp + Reactity Insertions/2(Xe Reactivity)
  (n/n_0)/1 -> Xe Reactivity/1(n0)
